simulink model "RCAM0_sim"  (R2023a)
settings: Solver=VariableStepAuto  StartTime=0.0  StopTime=TF  RelTol=1e-3
values from neighbouring files (symbols this model uses):
  u0 = [0 ... (first row only)    [RCAM0_init.m]    (also in RCAM_constants.mat = [0 -0.194874130949 0 0.0795600512836 0.0795600512836]; RCAM_dynamics.m = u; RCAM_init.m = deg2rad(u0); RCAM_init2.m = ustar)
  x0 = [85 ... (first row only)    [RCAM0_init.m]    (also in RCAM_trim1.m = [Vb0;pqr0;euler0;Xe0]; RCAM_trim1v2.m = [Va_target; RCAM_trim2.m = [Va_target)
undefined symbols (not defined in the file or in its folder): RCAM_model0
settings Model: Creator=Reggie Johanes  LastModifiedBy=Reggie Johanes

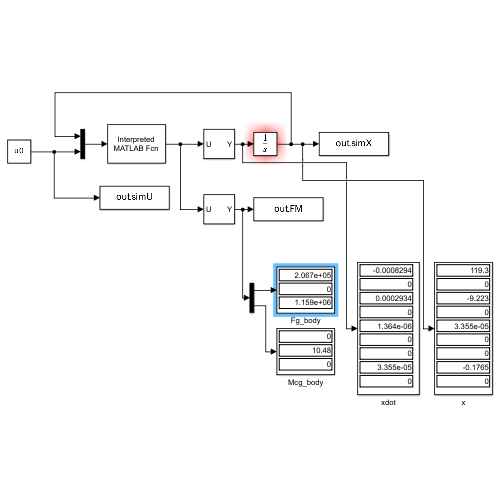
[thumbnail: Simulink's stored preview of the top-level diagram]
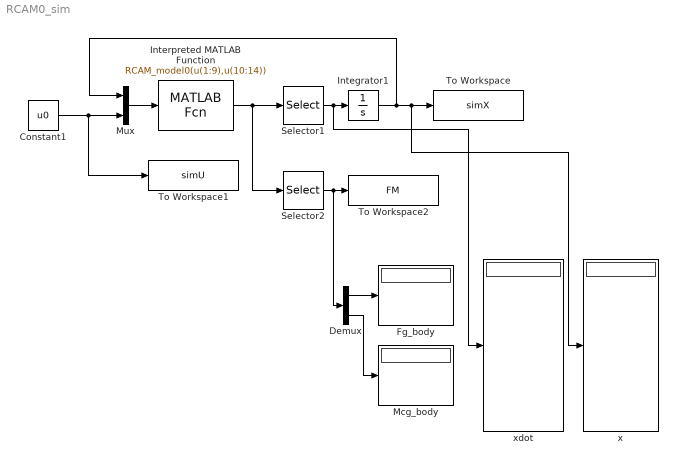
== system RCAM0_sim ==
  Constant1 : Constant  Value=u0
  Demux : Demux  Outputs=2
  Fg_body : Display
  Integrator1 : Integrator  InitialCondition=x0
  Interpreted MATLAB Function : MATLABFcn  MATLABFcn=RCAM_model0(u(1:9),u(10:14))
  Mcg_body : Display
  Mux : Mux  Inputs=2
  Selector1 : Selector  InputPortWidth=15  IndexOptions=Index vector (dialog)  Indices=[1:9]  OutputSizes=1
  Selector2 : Selector  InputPortWidth=15  IndexOptions=Index vector (dialog)  Indices=[10:15]  OutputSizes=1
  To Workspace : ToWorkspace  VariableName=simX  SaveFormat=Timeseries  SampleTime=-1
  To Workspace1 : ToWorkspace  VariableName=simU  SaveFormat=Timeseries  SampleTime=-1
  To Workspace2 : ToWorkspace  VariableName=FM  SaveFormat=Timeseries  SampleTime=-1
  x : Display
  xdot : Display
  wires:
  Mux/1 -> Interpreted MATLAB Function/1
  Constant1/1 -> To Workspace1/1, Mux/2
  Interpreted MATLAB Function/1 -> Selector2/1, Selector1/1
  Integrator1/1 -> x/1, To Workspace/1, Mux/1
  Selector1/1 -> Integrator1/1, xdot/1
  Selector2/1 -> Demux/1, To Workspace2/1
  Demux/2 -> Mcg_body/1
  Demux/1 -> Fg_body/1
